simulink model "TST_FuelT_DD"  (R2016b)
settings: Solver=FixedStepDiscrete  StartTime=0.0  StopTime=simTime  FixedStep=sampleTime  RelTol=1e-3
values from neighbouring files (symbols this model uses):
  testCase = 1    [initTST_FuelT_DD_001.m]
libraries: simulink x11, UnitTest_Lib x9
settings Model: Creator=zhengjinyan  LastModifiedBy=zhengjinyan
settings DebuggingCC: SignalRangeChecking=error

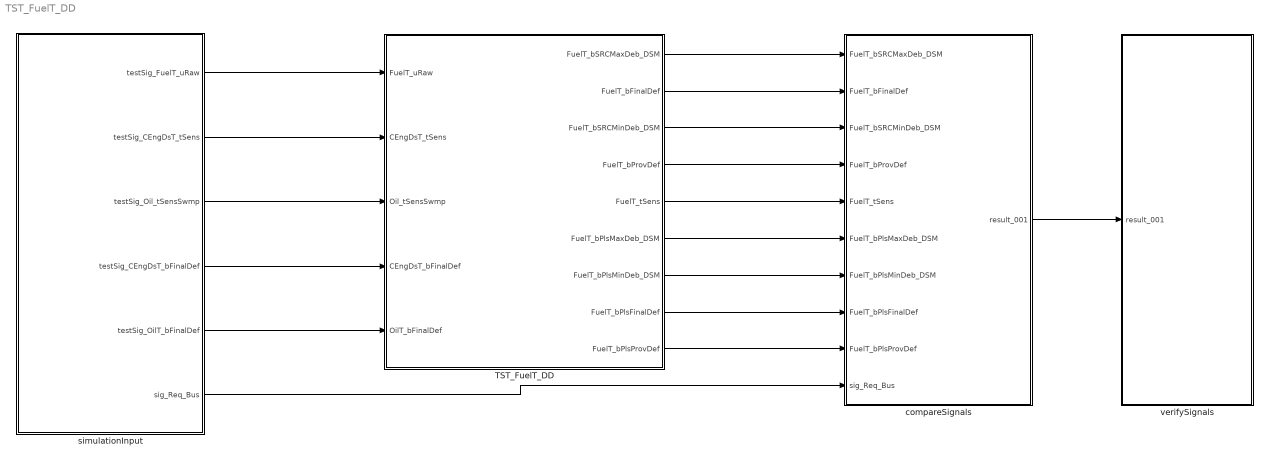
== system TST_FuelT_DD ==
  TST_FuelT_DD : Subsystem
  compareSignals : Subsystem
  simulationInput : Subsystem
  verifySignals : Subsystem
  wires:
  simulationInput/1(testSig_FuelT_uRaw) -> TST_FuelT_DD/1(FuelT_uRaw)
  simulationInput/2(testSig_CEngDsT_tSens) -> TST_FuelT_DD/2(CEngDsT_tSens)
  simulationInput/3(testSig_Oil_tSensSwmp) -> TST_FuelT_DD/3(Oil_tSensSwmp)
  simulationInput/4(testSig_CEngDsT_bFinalDef) -> TST_FuelT_DD/4(CEngDsT_bFinalDef)
  simulationInput/5(testSig_OilT_bFinalDef) -> TST_FuelT_DD/5(OilT_bFinalDef)
  TST_FuelT_DD/1(FuelT_bSRCMaxDeb_DSM) -> compareSignals/1(FuelT_bSRCMaxDeb_DSM)
  TST_FuelT_DD/2(FuelT_bFinalDef) -> compareSignals/2(FuelT_bFinalDef)
  TST_FuelT_DD/3(FuelT_bSRCMinDeb_DSM) -> compareSignals/3(FuelT_bSRCMinDeb_DSM)
  TST_FuelT_DD/4(FuelT_bProvDef) -> compareSignals/4(FuelT_bProvDef)
  TST_FuelT_DD/5(FuelT_tSens) -> compareSignals/5(FuelT_tSens)
  TST_FuelT_DD/6(FuelT_bPlsMaxDeb_DSM) -> compareSignals/6(FuelT_bPlsMaxDeb_DSM)
  TST_FuelT_DD/7(FuelT_bPlsMinDeb_DSM) -> compareSignals/7(FuelT_bPlsMinDeb_DSM)
  TST_FuelT_DD/8(FuelT_bPlsFinalDef) -> compareSignals/8(FuelT_bPlsFinalDef)
  TST_FuelT_DD/9(FuelT_bPlsProvDef) -> compareSignals/9(FuelT_bPlsProvDef)
  simulationInput/6(sig_Req_Bus) -> compareSignals/10(sig_Req_Bus)
  compareSignals/1(result_001) -> verifySignals/1(result_001)

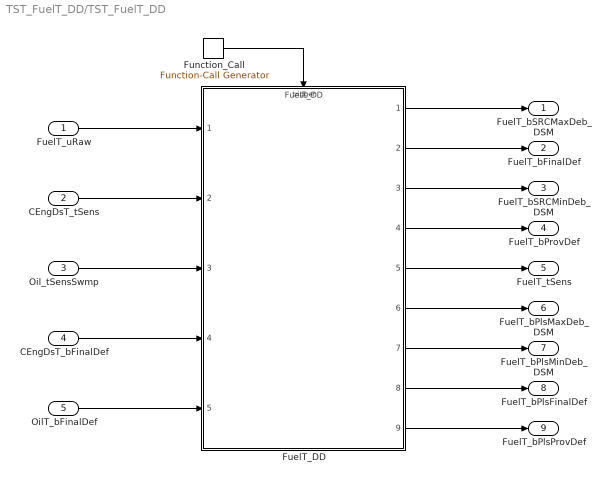
== system TST_FuelT_DD/TST_FuelT_DD ==
  FuelT_uRaw : Inport
  CEngDsT_tSens : Inport  Port=2
  Oil_tSensSwmp : Inport  Port=3
  CEngDsT_bFinalDef : Inport  Port=4
  OilT_bFinalDef : Inport  Port=5
  FuelT_DD : ModelReference  ModelNameDialog=FuelT_DD  SimulationMode=Normal  ModelReferenceVersion=1.4  TriggerPortName=function  TriggerPortTriggerType=function-call  TriggerPortStatesWhenEnabling=held
  Function_Call : simulink/Ports & Subsystems/Function-Call Generator  sample_time=sampleTime  numberOfIterations=1
  FuelT_bSRCMaxDeb_DSM : Outport
  FuelT_bFinalDef : Outport  Port=2
  FuelT_bSRCMinDeb_DSM : Outport  Port=3
  FuelT_bProvDef : Outport  Port=4
  FuelT_tSens : Outport  Port=5
  FuelT_bPlsMaxDeb_DSM : Outport  Port=6
  FuelT_bPlsMinDeb_DSM : Outport  Port=7
  FuelT_bPlsFinalDef : Outport  Port=8
  FuelT_bPlsProvDef : Outport  Port=9
  wires:
  Function_Call/1 -> FuelT_DD/Trigger
  FuelT_uRaw/1 -> FuelT_DD/1
  CEngDsT_tSens/1 -> FuelT_DD/2
  Oil_tSensSwmp/1 -> FuelT_DD/3
  CEngDsT_bFinalDef/1 -> FuelT_DD/4
  OilT_bFinalDef/1 -> FuelT_DD/5
  FuelT_DD/1 -> FuelT_bSRCMaxDeb_DSM/1
  FuelT_DD/2 -> FuelT_bFinalDef/1
  FuelT_DD/3 -> FuelT_bSRCMinDeb_DSM/1
  FuelT_DD/4 -> FuelT_bProvDef/1
  FuelT_DD/5 -> FuelT_tSens/1
  FuelT_DD/6 -> FuelT_bPlsMaxDeb_DSM/1
  FuelT_DD/7 -> FuelT_bPlsMinDeb_DSM/1
  FuelT_DD/8 -> FuelT_bPlsFinalDef/1
  FuelT_DD/9 -> FuelT_bPlsProvDef/1

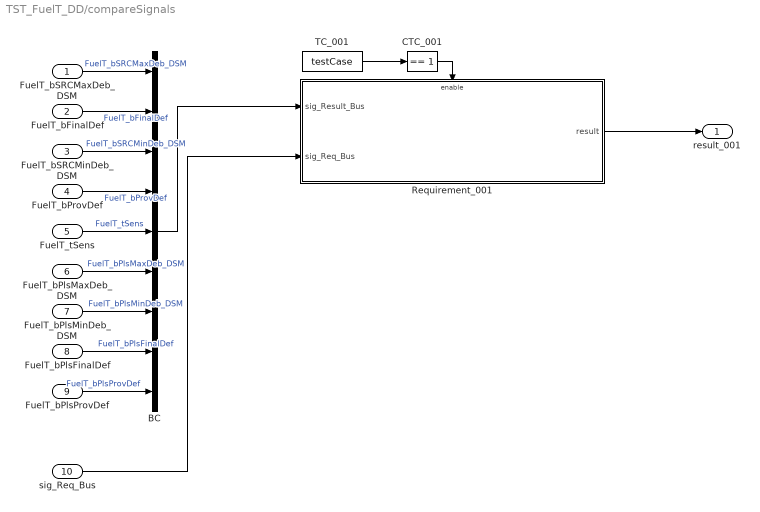
== system TST_FuelT_DD/compareSignals ==
  FuelT_bSRCMaxDeb_DSM : Inport
  FuelT_bFinalDef : Inport  Port=2
  FuelT_bSRCMinDeb_DSM : Inport  Port=3
  FuelT_bProvDef : Inport  Port=4
  FuelT_tSens : Inport  Port=5
  FuelT_bPlsMaxDeb_DSM : Inport  Port=6
  FuelT_bPlsMinDeb_DSM : Inport  Port=7
  FuelT_bPlsFinalDef : Inport  Port=8
  FuelT_bPlsProvDef : Inport  Port=9
  sig_Req_Bus : Inport  Port=10
  BC : BusCreator  Inputs=9
  CTC_001 : simulink/Logic and Bit Operations/Compare To Constant  relop===  const=1  OutDataTypeStr=boolean
  Requirement_001 : Subsystem
  TC_001 : Constant  Value=testCase
  result_001 : Outport
  wires:
  FuelT_bSRCMaxDeb_DSM/1 -> BC/1  "FuelT_bSRCMaxDeb_DSM"
  FuelT_bFinalDef/1 -> BC/2  "FuelT_bFinalDef"
  FuelT_bSRCMinDeb_DSM/1 -> BC/3  "FuelT_bSRCMinDeb_DSM"
  FuelT_bProvDef/1 -> BC/4  "FuelT_bProvDef"
  FuelT_tSens/1 -> BC/5  "FuelT_tSens"
  FuelT_bPlsMaxDeb_DSM/1 -> BC/6  "FuelT_bPlsMaxDeb_DSM"
  FuelT_bPlsMinDeb_DSM/1 -> BC/7  "FuelT_bPlsMinDeb_DSM"
  FuelT_bPlsFinalDef/1 -> BC/8  "FuelT_bPlsFinalDef"
  FuelT_bPlsProvDef/1 -> BC/9  "FuelT_bPlsProvDef"
  TC_001/1 -> CTC_001/1
  CTC_001/1 -> Requirement_001/Enable
  sig_Req_Bus/1 -> Requirement_001/2(sig_Req_Bus)
  BC/1 -> Requirement_001/1(sig_Result_Bus)
  Requirement_001/1(result) -> result_001/1

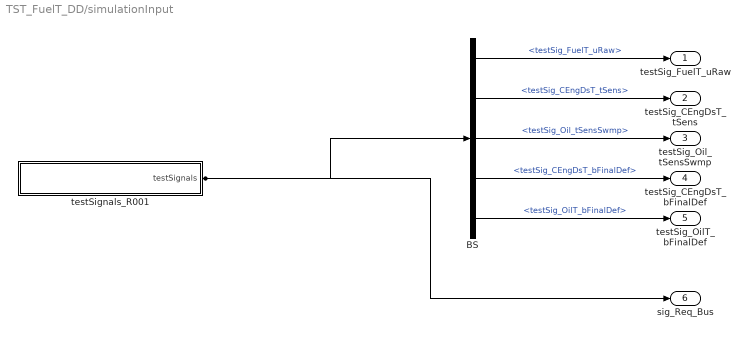
== system TST_FuelT_DD/simulationInput ==
  BS : BusSelector  OutputSignals=testSig_FuelT_uRaw,testSig_CEngDsT_tSens,testSig_Oil_tSensSwmp,testSig_CEngDsT_bFinalDef,testSig_OilT_bFinalDef
  testSignals_R001 : Subsystem
  testSig_FuelT_uRaw : Outport
  testSig_CEngDsT_tSens : Outport  Port=2
  testSig_Oil_tSensSwmp : Outport  Port=3
  testSig_CEngDsT_bFinalDef : Outport  Port=4
  testSig_OilT_bFinalDef : Outport  Port=5
  sig_Req_Bus : Outport  Port=6
  wires:
  BS/1 -> testSig_FuelT_uRaw/1  "<testSig_FuelT_uRaw>"
  BS/2 -> testSig_CEngDsT_tSens/1  "<testSig_CEngDsT_tSens>"
  BS/3 -> testSig_Oil_tSensSwmp/1  "<testSig_Oil_tSensSwmp>"
  BS/4 -> testSig_CEngDsT_bFinalDef/1  "<testSig_CEngDsT_bFinalDef>"
  BS/5 -> testSig_OilT_bFinalDef/1  "<testSig_OilT_bFinalDef>"
  testSignals_R001/1(testSignals) -> BS/1, sig_Req_Bus/1

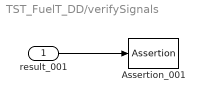
== system TST_FuelT_DD/verifySignals ==
  result_001 : Inport
  Assertion_001 : Assertion  Enabled=off
  wires:
  result_001/1 -> Assertion_001/1

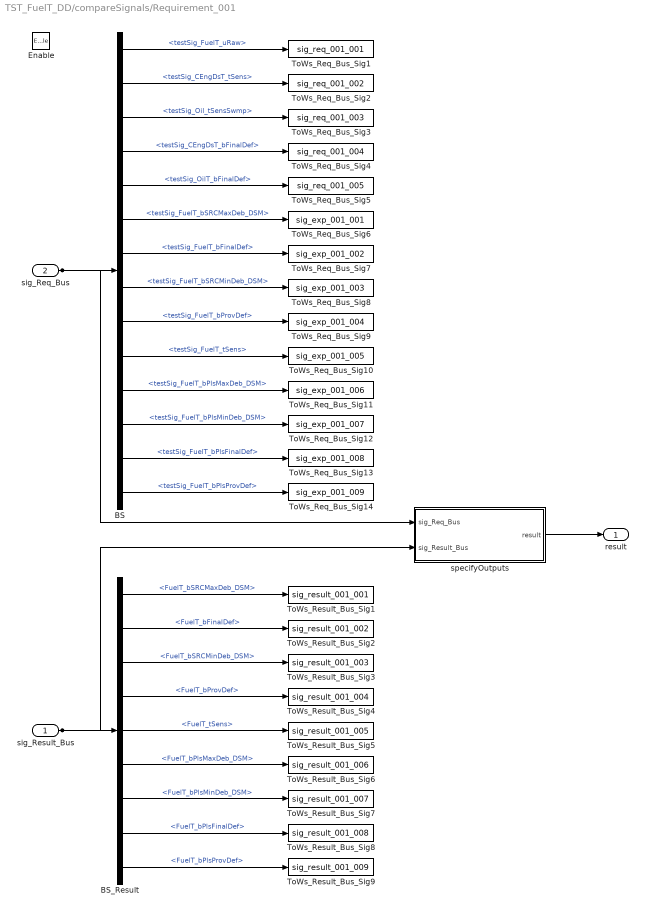
== system TST_FuelT_DD/compareSignals/Requirement_001 ==
  sig_Result_Bus : Inport
  sig_Req_Bus : Inport  Port=2
  Enable : EnablePort
  BS : BusSelector  OutputSignals=testSig_FuelT_uRaw,testSig_CEngDsT_tSens,testSig_Oil_tSensSwmp,testSig_CEngDsT_bFinalDef,testSig_OilT_bFinalDef,testSig_FuelT_bSRCMaxDeb_DSM,testSig_FuelT_bFinalDef,testSig_FuelT_bSRCMinDeb_DSM,testSig_FuelT_bProvDef,testSig_FuelT_tSens,testSig_FuelT_bPlsMaxDeb_DSM,testSig_FuelT_bPlsMinDeb_DSM,testSig_FuelT_bPlsFinalDef,testSig_FuelT_bPlsProvDef
  BS_Result : BusSelector  OutputSignals=FuelT_bSRCMaxDeb_DSM,FuelT_bFinalDef,FuelT_bSRCMinDeb_DSM,FuelT_bProvDef,FuelT_tSens,FuelT_bPlsMaxDeb_DSM,FuelT_bPlsMinDeb_DSM,FuelT_bPlsFinalDef,FuelT_bPlsProvDef
  ToWs_Req_Bus_Sig1 : ToWorkspace  VariableName=sig_req_001_001  SaveFormat=Structure With Time
  ToWs_Req_Bus_Sig10 : ToWorkspace  VariableName=sig_exp_001_005  SaveFormat=Structure With Time
  ToWs_Req_Bus_Sig11 : ToWorkspace  VariableName=sig_exp_001_006  SaveFormat=Structure With Time
  ToWs_Req_Bus_Sig12 : ToWorkspace  VariableName=sig_exp_001_007  SaveFormat=Structure With Time
  ToWs_Req_Bus_Sig13 : ToWorkspace  VariableName=sig_exp_001_008  SaveFormat=Structure With Time
  ToWs_Req_Bus_Sig14 : ToWorkspace  VariableName=sig_exp_001_009  SaveFormat=Structure With Time
  ToWs_Req_Bus_Sig2 : ToWorkspace  VariableName=sig_req_001_002  SaveFormat=Structure With Time
  ToWs_Req_Bus_Sig3 : ToWorkspace  VariableName=sig_req_001_003  SaveFormat=Structure With Time
  ToWs_Req_Bus_Sig4 : ToWorkspace  VariableName=sig_req_001_004  SaveFormat=Structure With Time
  ToWs_Req_Bus_Sig5 : ToWorkspace  VariableName=sig_req_001_005  SaveFormat=Structure With Time
  ToWs_Req_Bus_Sig6 : ToWorkspace  VariableName=sig_exp_001_001  SaveFormat=Structure With Time
  ToWs_Req_Bus_Sig7 : ToWorkspace  VariableName=sig_exp_001_002  SaveFormat=Structure With Time
  ToWs_Req_Bus_Sig8 : ToWorkspace  VariableName=sig_exp_001_003  SaveFormat=Structure With Time
  ToWs_Req_Bus_Sig9 : ToWorkspace  VariableName=sig_exp_001_004  SaveFormat=Structure With Time
  ToWs_Result_Bus_Sig1 : ToWorkspace  VariableName=sig_result_001_001  SaveFormat=Structure With Time
  ToWs_Result_Bus_Sig2 : ToWorkspace  VariableName=sig_result_001_002  SaveFormat=Structure With Time
  ToWs_Result_Bus_Sig3 : ToWorkspace  VariableName=sig_result_001_003  SaveFormat=Structure With Time
  ToWs_Result_Bus_Sig4 : ToWorkspace  VariableName=sig_result_001_004  SaveFormat=Structure With Time
  ToWs_Result_Bus_Sig5 : ToWorkspace  VariableName=sig_result_001_005  SaveFormat=Structure With Time
  ToWs_Result_Bus_Sig6 : ToWorkspace  VariableName=sig_result_001_006  SaveFormat=Structure With Time
  ToWs_Result_Bus_Sig7 : ToWorkspace  VariableName=sig_result_001_007  SaveFormat=Structure With Time
  ToWs_Result_Bus_Sig8 : ToWorkspace  VariableName=sig_result_001_008  SaveFormat=Structure With Time
  ToWs_Result_Bus_Sig9 : ToWorkspace  VariableName=sig_result_001_009  SaveFormat=Structure With Time
  specifyOutputs : Subsystem
  result : Outport
  wires:
  sig_Req_Bus/1 -> BS/1, specifyOutputs/1(sig_Req_Bus)
  BS/1 -> ToWs_Req_Bus_Sig1/1  "<testSig_FuelT_uRaw>"
  BS/2 -> ToWs_Req_Bus_Sig2/1  "<testSig_CEngDsT_tSens>"
  BS/3 -> ToWs_Req_Bus_Sig3/1  "<testSig_Oil_tSensSwmp>"
  BS/4 -> ToWs_Req_Bus_Sig4/1  "<testSig_CEngDsT_bFinalDef>"
  BS/5 -> ToWs_Req_Bus_Sig5/1  "<testSig_OilT_bFinalDef>"
  BS/6 -> ToWs_Req_Bus_Sig6/1  "<testSig_FuelT_bSRCMaxDeb_DSM>"
  BS/7 -> ToWs_Req_Bus_Sig7/1  "<testSig_FuelT_bFinalDef>"
  BS/8 -> ToWs_Req_Bus_Sig8/1  "<testSig_FuelT_bSRCMinDeb_DSM>"
  BS/9 -> ToWs_Req_Bus_Sig9/1  "<testSig_FuelT_bProvDef>"
  BS/10 -> ToWs_Req_Bus_Sig10/1  "<testSig_FuelT_tSens>"
  BS/11 -> ToWs_Req_Bus_Sig11/1  "<testSig_FuelT_bPlsMaxDeb_DSM>"
  BS/12 -> ToWs_Req_Bus_Sig12/1  "<testSig_FuelT_bPlsMinDeb_DSM>"
  BS/13 -> ToWs_Req_Bus_Sig13/1  "<testSig_FuelT_bPlsFinalDef>"
  BS/14 -> ToWs_Req_Bus_Sig14/1  "<testSig_FuelT_bPlsProvDef>"
  sig_Result_Bus/1 -> BS_Result/1, specifyOutputs/2(sig_Result_Bus)
  BS_Result/1 -> ToWs_Result_Bus_Sig1/1  "<FuelT_bSRCMaxDeb_DSM>"
  BS_Result/2 -> ToWs_Result_Bus_Sig2/1  "<FuelT_bFinalDef>"
  BS_Result/3 -> ToWs_Result_Bus_Sig3/1  "<FuelT_bSRCMinDeb_DSM>"
  BS_Result/4 -> ToWs_Result_Bus_Sig4/1  "<FuelT_bProvDef>"
  BS_Result/5 -> ToWs_Result_Bus_Sig5/1  "<FuelT_tSens>"
  BS_Result/6 -> ToWs_Result_Bus_Sig6/1  "<FuelT_bPlsMaxDeb_DSM>"
  BS_Result/7 -> ToWs_Result_Bus_Sig7/1  "<FuelT_bPlsMinDeb_DSM>"
  BS_Result/8 -> ToWs_Result_Bus_Sig8/1  "<FuelT_bPlsFinalDef>"
  BS_Result/9 -> ToWs_Result_Bus_Sig9/1  "<FuelT_bPlsProvDef>"
  specifyOutputs/1(result) -> result/1

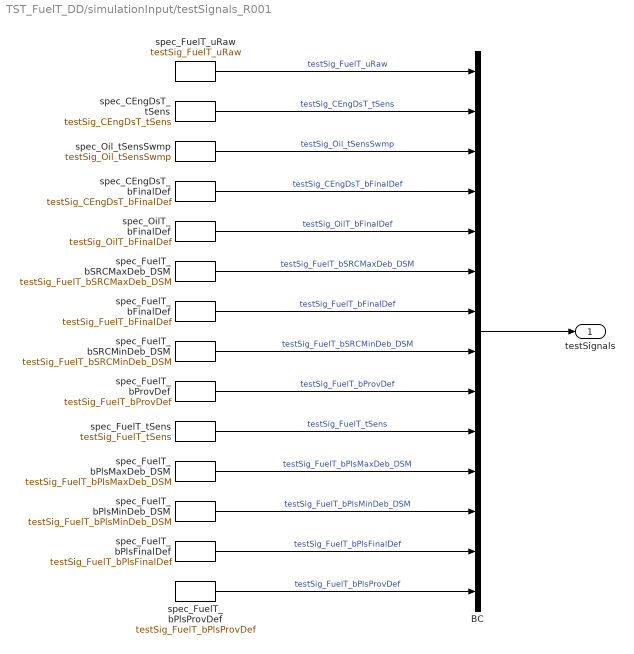
== system TST_FuelT_DD/simulationInput/testSignals_R001 ==
  BC : BusCreator  Inputs=14
  spec_CEngDsT_bFinalDef : FromWorkspace  VariableName=testSig_CEngDsT_bFinalDef  Interpolate=off  OutputAfterFinalValue=Holding final value
  spec_CEngDsT_tSens : FromWorkspace  VariableName=testSig_CEngDsT_tSens  Interpolate=off  OutputAfterFinalValue=Holding final value
  spec_FuelT_bFinalDef : FromWorkspace  VariableName=testSig_FuelT_bFinalDef  Interpolate=off  OutputAfterFinalValue=Holding final value
  spec_FuelT_bPlsFinalDef : FromWorkspace  VariableName=testSig_FuelT_bPlsFinalDef  Interpolate=off  OutputAfterFinalValue=Holding final value
  spec_FuelT_bPlsMaxDeb_DSM : FromWorkspace  VariableName=testSig_FuelT_bPlsMaxDeb_DSM  Interpolate=off  OutputAfterFinalValue=Holding final value
  spec_FuelT_bPlsMinDeb_DSM : FromWorkspace  VariableName=testSig_FuelT_bPlsMinDeb_DSM  Interpolate=off  OutputAfterFinalValue=Holding final value
  spec_FuelT_bPlsProvDef : FromWorkspace  VariableName=testSig_FuelT_bPlsProvDef  Interpolate=off  OutputAfterFinalValue=Holding final value
  spec_FuelT_bProvDef : FromWorkspace  VariableName=testSig_FuelT_bProvDef  Interpolate=off  OutputAfterFinalValue=Holding final value
  spec_FuelT_bSRCMaxDeb_DSM : FromWorkspace  VariableName=testSig_FuelT_bSRCMaxDeb_DSM  Interpolate=off  OutputAfterFinalValue=Holding final value
  spec_FuelT_bSRCMinDeb_DSM : FromWorkspace  VariableName=testSig_FuelT_bSRCMinDeb_DSM  Interpolate=off  OutputAfterFinalValue=Holding final value
  spec_FuelT_tSens : FromWorkspace  VariableName=testSig_FuelT_tSens  Interpolate=off  OutputAfterFinalValue=Holding final value
  spec_FuelT_uRaw : FromWorkspace  VariableName=testSig_FuelT_uRaw  Interpolate=off  OutputAfterFinalValue=Holding final value
  spec_OilT_bFinalDef : FromWorkspace  VariableName=testSig_OilT_bFinalDef  Interpolate=off  OutputAfterFinalValue=Holding final value
  spec_Oil_tSensSwmp : FromWorkspace  VariableName=testSig_Oil_tSensSwmp  Interpolate=off  OutputAfterFinalValue=Holding final value
  testSignals : Outport
  wires:
  BC/1 -> testSignals/1
  spec_FuelT_uRaw/1 -> BC/1  "testSig_FuelT_uRaw"
  spec_CEngDsT_tSens/1 -> BC/2  "testSig_CEngDsT_tSens"
  spec_Oil_tSensSwmp/1 -> BC/3  "testSig_Oil_tSensSwmp"
  spec_CEngDsT_bFinalDef/1 -> BC/4  "testSig_CEngDsT_bFinalDef"
  spec_OilT_bFinalDef/1 -> BC/5  "testSig_OilT_bFinalDef"
  spec_FuelT_bSRCMaxDeb_DSM/1 -> BC/6  "testSig_FuelT_bSRCMaxDeb_DSM"
  spec_FuelT_bFinalDef/1 -> BC/7  "testSig_FuelT_bFinalDef"
  spec_FuelT_bSRCMinDeb_DSM/1 -> BC/8  "testSig_FuelT_bSRCMinDeb_DSM"
  spec_FuelT_bProvDef/1 -> BC/9  "testSig_FuelT_bProvDef"
  spec_FuelT_tSens/1 -> BC/10  "testSig_FuelT_tSens"
  spec_FuelT_bPlsMaxDeb_DSM/1 -> BC/11  "testSig_FuelT_bPlsMaxDeb_DSM"
  spec_FuelT_bPlsMinDeb_DSM/1 -> BC/12  "testSig_FuelT_bPlsMinDeb_DSM"
  spec_FuelT_bPlsFinalDef/1 -> BC/13  "testSig_FuelT_bPlsFinalDef"
  spec_FuelT_bPlsProvDef/1 -> BC/14  "testSig_FuelT_bPlsProvDef"

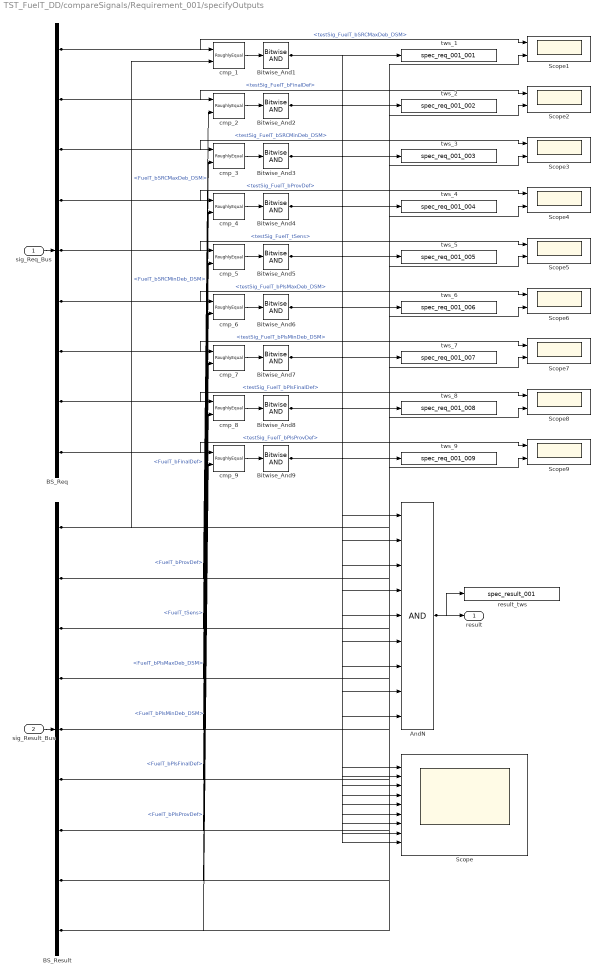
== system TST_FuelT_DD/compareSignals/Requirement_001/specifyOutputs ==
  sig_Req_Bus : Inport
  sig_Result_Bus : Inport  Port=2
  AndN : Logic  Inputs=9
  BS_Req : BusSelector  OutputSignals=testSig_FuelT_bSRCMaxDeb_DSM,testSig_FuelT_bFinalDef,testSig_FuelT_bSRCMinDeb_DSM,testSig_FuelT_bProvDef,testSig_FuelT_tSens,testSig_FuelT_bPlsMaxDeb_DSM,testSig_FuelT_bPlsMinDeb_DSM,testSig_FuelT_bPlsFinalDef,testSig_FuelT_bPlsProvDef
  BS_Result : BusSelector  OutputSignals=FuelT_bSRCMaxDeb_DSM,FuelT_bFinalDef,FuelT_bSRCMinDeb_DSM,FuelT_bProvDef,FuelT_tSens,FuelT_bPlsMaxDeb_DSM,FuelT_bPlsMinDeb_DSM,FuelT_bPlsFinalDef,FuelT_bPlsProvDef
  Bitwise_And{1..9} (9 alike) : simulink/Logic and Bit Operations/Bitwise Operator  logicop=AND  UseBitMask=off  BitMask=bin2dec('11011001')  BitMaskRealWorld=Stored Integer
  Scope : Scope  NumInputPorts=9
  Scope{1..9} (9 alike) : Scope  NumInputPorts=2
  cmp_{1..9} (9 alike) : UnitTest_Lib/RoughlyEqual  slope=0.1
  result_tws : ToWorkspace  VariableName=spec_result_001
  tws_1 : ToWorkspace  VariableName=spec_req_001_001
  tws_2 : ToWorkspace  VariableName=spec_req_001_002
  tws_3 : ToWorkspace  VariableName=spec_req_001_003
  tws_4 : ToWorkspace  VariableName=spec_req_001_004
  tws_5 : ToWorkspace  VariableName=spec_req_001_005
  tws_6 : ToWorkspace  VariableName=spec_req_001_006
  tws_7 : ToWorkspace  VariableName=spec_req_001_007
  tws_8 : ToWorkspace  VariableName=spec_req_001_008
  tws_9 : ToWorkspace  VariableName=spec_req_001_009
  result : Outport
  wires:
  sig_Req_Bus/1 -> BS_Req/1
  sig_Result_Bus/1 -> BS_Result/1
  AndN/1 -> result/1, result_tws/1
  BS_Req/1 -> cmp_1/1, Scope1/1  "<testSig_FuelT_bSRCMaxDeb_DSM>"
  BS_Result/1 -> cmp_1/2, Scope1/2  "<FuelT_bSRCMaxDeb_DSM>"
  cmp_1/1 -> Bitwise_And1/1
  Bitwise_And1/1 -> tws_1/1, AndN/1, Scope/1
  BS_Req/2 -> cmp_2/1, Scope2/1  "<testSig_FuelT_bFinalDef>"
  BS_Result/2 -> cmp_2/2, Scope2/2  "<FuelT_bFinalDef>"
  cmp_2/1 -> Bitwise_And2/1
  Bitwise_And2/1 -> tws_2/1, AndN/2, Scope/2
  BS_Req/3 -> cmp_3/1, Scope3/1  "<testSig_FuelT_bSRCMinDeb_DSM>"
  BS_Result/3 -> cmp_3/2, Scope3/2  "<FuelT_bSRCMinDeb_DSM>"
  cmp_3/1 -> Bitwise_And3/1
  Bitwise_And3/1 -> tws_3/1, AndN/3, Scope/3
  BS_Req/4 -> cmp_4/1, Scope4/1  "<testSig_FuelT_bProvDef>"
  BS_Result/4 -> cmp_4/2, Scope4/2  "<FuelT_bProvDef>"
  cmp_4/1 -> Bitwise_And4/1
  Bitwise_And4/1 -> tws_4/1, AndN/4, Scope/4
  BS_Req/5 -> cmp_5/1, Scope5/1  "<testSig_FuelT_tSens>"
  BS_Result/5 -> cmp_5/2, Scope5/2  "<FuelT_tSens>"
  cmp_5/1 -> Bitwise_And5/1
  Bitwise_And5/1 -> tws_5/1, AndN/5, Scope/5
  BS_Req/6 -> cmp_6/1, Scope6/1  "<testSig_FuelT_bPlsMaxDeb_DSM>"
  BS_Result/6 -> cmp_6/2, Scope6/2  "<FuelT_bPlsMaxDeb_DSM>"
  cmp_6/1 -> Bitwise_And6/1
  Bitwise_And6/1 -> tws_6/1, AndN/6, Scope/6
  BS_Req/7 -> cmp_7/1, Scope7/1  "<testSig_FuelT_bPlsMinDeb_DSM>"
  BS_Result/7 -> cmp_7/2, Scope7/2  "<FuelT_bPlsMinDeb_DSM>"
  cmp_7/1 -> Bitwise_And7/1
  Bitwise_And7/1 -> tws_7/1, AndN/7, Scope/7
  BS_Req/8 -> cmp_8/1, Scope8/1  "<testSig_FuelT_bPlsFinalDef>"
  BS_Result/8 -> cmp_8/2, Scope8/2  "<FuelT_bPlsFinalDef>"
  cmp_8/1 -> Bitwise_And8/1
  Bitwise_And8/1 -> tws_8/1, AndN/8, Scope/8
  BS_Req/9 -> cmp_9/1, Scope9/1  "<testSig_FuelT_bPlsProvDef>"
  BS_Result/9 -> cmp_9/2, Scope9/2  "<FuelT_bPlsProvDef>"
  cmp_9/1 -> Bitwise_And9/1
  Bitwise_And9/1 -> tws_9/1, AndN/9, Scope/9
